simulink model "FullSystemCyclesv4"  (R2020b)
settings: Solver=FixedStepAuto  StartTime=0.0  StopTime=1800  FixedStep=0.005  RelTol=1e-3
libraries: fl_lib x34, nesl_utility x20, SimscapeFluids_lib x6, slpidlib x1
(part 2 of 2)

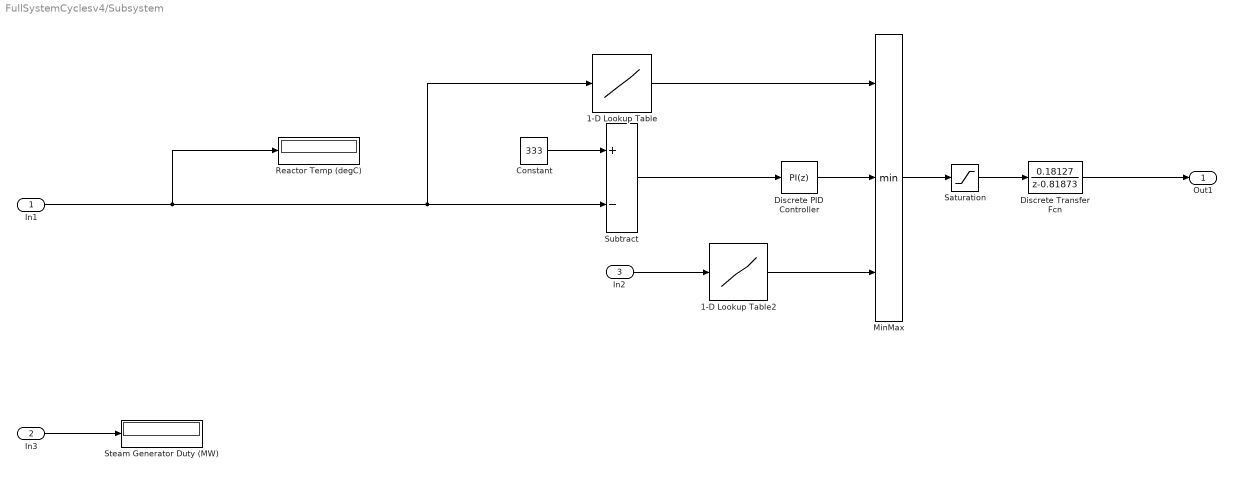
== system FullSystemCyclesv4/Subsystem ==
  In1 : Inport
  In3 : Inport  Port=2
  In2 : Inport  Port=3
  1-D Lookup Table : Lookup_n-D  NumberOfTableDimensions=1  BreakpointsForDimension1=[315 320 325 330 332 333 334 335]  Table=[3.0 2.5 2.0 1.5 1.2 1.0 0.6 0]  InternalRulePriority=Speed  RndMeth=Simplest  InputSameDT=on
  1-D Lookup Table2 : Lookup_n-D  NumberOfTableDimensions=1  BreakpointsForDimension1=[0.00 0.80 0.85 0.90 0.93 0.95 0.97 0.98 0.99 1.00]  Table=[3.0 3.0 3.0 2.9 2.7 2.4 1.8 1.2 0.5 0]  ExtrapMethod=Clip  DiagnosticForOutOfRangeInput=Warning  UseLastTableValue=on  InternalRulePriority=Speed  RndMeth=Simplest  InputSameDT=on
  Constant : Constant  Value=333
  Discrete Transfer Fcn : DiscreteTransferFcn  Numerator=[0.18127]  Denominator=[1 -0.81873]  SampleTime=0.005
  Discrete PID Controller : slpidlib/PID Controller  Controller=PI  Form=Parallel  TimeDomain=Discrete-time  UseExternalTs=off  SampleTime=0.005  IntegratorMethod=Forward Euler  FilterMethod=Forward Euler  ControllerParametersSource=internal  P=0.01  I=0.002  D=0  UseFilter=on  N=100  TunerSelectOption=Transfer Function Based (PID Tuner App)  InitialConditionSource=internal  InitialConditionForIntegrator=0.5  InitialConditionForFilter=0  DifferentiatorICPrevScaledInput=0  ExternalReset=none  TrackingMode=off  Kt=1  LimitOutput=on  SatLimitsSource=internal  UpperSaturationLimit=3  LowerSaturationLimit=0  LinearizeAsGain=off  AntiWindupMode=clamping  Kb=1  POutMin=[]  POutMax=[]  IOutMin=[]  IOutMax=[]  DOutMin=[]  DOutMax=[]  NOutMin=[]  NOutMax=[]  SumOutMin=[]  SumOutMax=[]  SaturationOutMin=[]  SaturationOutMax=[]  PParamMin=[]  PParamMax=[]  IParamMin=[]  IParamMax=[]  DParamMin=[]  DParamMax=[]  NParamMin=[]  NParamMax=[]  KbParamMin=[]  KbParamMax=[]  KtParamMin=[]  KtParamMax=[]  KbOutMin=[]  KbOutMax=[]  KtOutMin=[]  KtOutMax=[]  IntegratorOutMin=[]  IntegratorOutMax=[]  FilterOutMin=[]  FilterOutMax=[]  SumI1OutMin=[]  SumI1OutMax=[]  SumI2OutMin=[]  SumI2OutMax=[]  SumI3OutMin=[]  SumI3OutMax=[]  SumI4OutMin=[]  SumI4OutMax=[]  SumDOutMin=[]  SumDOutMax=[]  DifferentiatorOutMin=[]  DifferentiatorOutMax=[]  FilterDiffOutCoefMin=[]  FilterDiffOutCoefMax=[]  ReciprocalOutMin=[]  ReciprocalOutMax=[]  SumDenOutMin=[]  SumDenOutMax=[]  SumNumOutMin=[]  SumNumOutMax=[]  DivideOutMin=[]  DivideOutMax=[]  UdiffTsProdOutMin=[]  UdiffTsProdOutMax=[]  NTsProdOutMin=[]  NTsProdOutMax=[]  UintegralTsProdOutMin=[]  UintegralTsProdOutMax=[]  UngainTsProdOutMin=[]  UngainTsProdOutMax=[]  IntegratorContinuousStateAttributes=''  IntegratorStateMustResolveToSignalObject=off  IntegratorRTWStateStorageClass=Auto  FilterContinuousStateAttributes=''  FilterStateMustResolveToSignalObject=off  FilterRTWStateStorageClass=Auto  ParallelPVariant=InternalParameters  IdealPVariant=Disabled  IVariant=InternalParameters  DVariant=Disabled  IntegratorVariant=Discrete  SatVariant=Enabled  AWVariant=DiscClampingParallel  PCopyVariant=Disabled  TRVariant=Disabled  FdbkBlocksVariant=Forward  IdealPFdbkVariant=Disabled  SatFdbkVariant=Disabled  DerivativeFilterVariant=Disabled  NVariant=Disabled  NCopyVariant=Disabled_SignalSpec  FilterICVariant=Disabled  IntegratorICVariant=InternalICs  ExternalResetVariant=Disabled  TRSumVariant=Passthrough  SumFdbkVariant=Disabled  SumVariant=Sum_PI  TsampFilterVariant=InternalTs  TsampNgainVariant=Passthrough  TsampIntegralVariant=Passthrough  ExternalSaturationOutDataTypeStr=Inherit: Same as second input
  MinMax : MinMax  Inputs=3
  Reactor Temp (degC) : Display
  Saturation : Saturate  UpperLimit=inf  LowerLimit=0
  Steam Generator Duty (MW) : Display
  Subtract : Sum  Inputs=+-
  Out1 : Outport
  wires:
  In1/1 -> Reactor Temp (degC)/1, 1-D Lookup Table/1, Subtract/2
  In3/1 -> Steam Generator Duty (MW)/1
  Constant/1 -> Subtract/1
  Subtract/1 -> Discrete PID Controller/1
  1-D Lookup Table/1 -> MinMax/1
  Discrete PID Controller/1 -> MinMax/2
  MinMax/1 -> Saturation/1
  Saturation/1 -> Discrete Transfer Fcn/1
  Discrete Transfer Fcn/1 -> Out1/1
  In2/1 -> 1-D Lookup Table2/1
  1-D Lookup Table2/1 -> MinMax/3
